simulink model "three_phase_squirrel_machine"  (R2017a)
settings: Solver=ode23tb  StartTime=0.0  StopTime=16  FixedStep=0.001  MaxStep=1e-4  MinStep=1e-7  RelTol=1e-3  AbsTol=.05  EnableMultiTasking=on
libraries: powerlib x17, simulink x1
settings Model: Creator=Administrator  LastModifiedBy=90584
settings DataIOCC: LimitDataPoints=on  SaveFormat=Array  SignalLoggingSaveFormat=ModelDataLogs
settings OptimizationCC: InitFltsAndDblsToZero=on  LifeSpan=inf
settings DebuggingCC: SaveWithParameterizedLinksMsg=none  UnderspecifiedInitializationDetection=Classic  MergeDetectMultiDrivingBlocksExec=none  SignalResolutionControl=TryResolveAllWithWarning  SolverPrmCheckMsg=warning  MultiTaskDSMMsg=warning  MultiTaskCondExecSysMsg=none  FcnCallInpInsideContextMsg=warning  SFUnexpectedBacktrackingDiag=warning  SFNoUnconditionalDefaultTransitionDiag=warning  SFExecutionAtInitializationDiag=none
settings HardwareCC: ProdBitPerPointer=32  ProdBitPerSizeT=32  ProdBitPerPtrDiffT=32  ProdLargestAtomicFloat=None  ProdIntDivRoundTo=Undefined  ProdEndianess=Unspecified  ProdWordSize=32  ProdHWDeviceType=32-bit Generic
settings ModelReferenceCC: PropagateSignalLabelsOutOfModel=off
settings GRTTargetCC: TargetFcnLib=ansi_tfl_tmw.mat  TargetLangStandard=C89/C90 (ANSI)  CombineOutputUpdateFcns=off  GRTInterface=on
settings ConfigComp: CovMetricSettings=dw  CovHtmlReporting=on  CovSaveCumulativeToWorkspaceVar=on  CovSaveSingleToWorkspaceVar=on  CovExternalEMLEnable=off

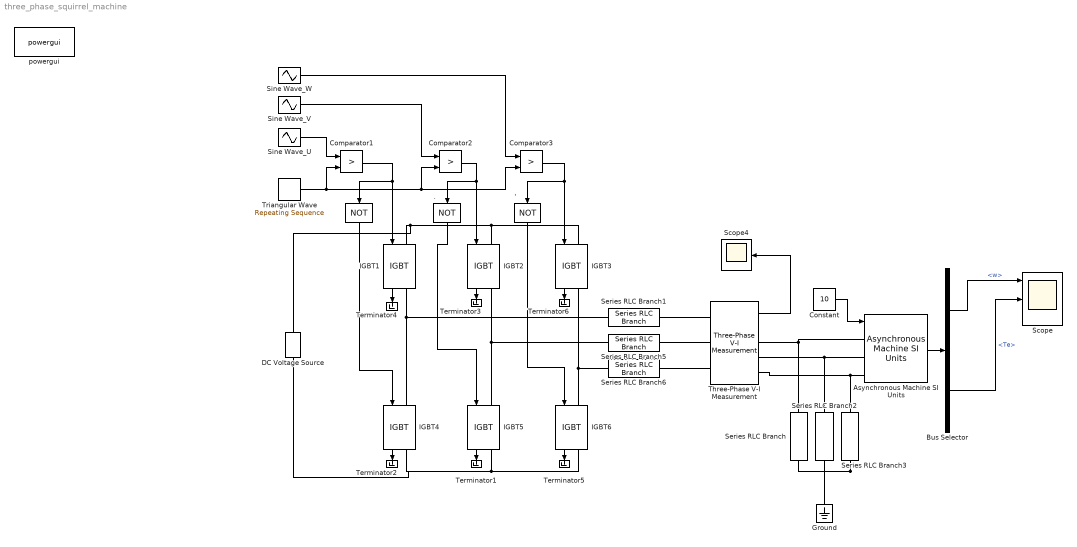
== system three_phase_squirrel_machine ==
  " " : Logic  Operator=NOT  AllPortsSameDT=off  OutDataTypeStr=boolean
  " '" : Logic  Operator=NOT  AllPortsSameDT=off  OutDataTypeStr=boolean
  " ." : Logic  Operator=NOT  AllPortsSameDT=off  OutDataTypeStr=boolean
  Asynchronous Machine SI Units : powerlib/Machines/Asynchronous Machine SI Units  RotorType=Squirrel-cage  PresetModel=No  MechanicalLoad=Torque Tm  ShowDetailedParameters=on  ReferenceFrame=Stationary  Units=SI  MeasurementBus=on  NominalParameters=[3*800,110,50]  Stator=[0.635 1*2.0e-3]  Rotor=[0.816 1.5e-3]  Cage1=[0.4155 0.002066]  Cage2=[0.4168 0.0003495]  Lm=76.31e-3  Mechanical=[0.25 0 2]  PolePairs=2  InitialConditions=[1 0 0 0 0 0 0 0]  SimulateSaturation=off  Saturation=[14.03593122, 27.81365428, 53.79336849, 72.68890987, 97.98006896, 148.6815601, 215.7428561, 302.9841135, 428.7778367 ; 230, 322, 414, 460, 506, 552, 598, 644, 690]  LoadFlowParameters=1492000  TsPowergui=0  TsBlock=-1  IterativeModel=Trapezoidal non iterative  IterativeDiscreteModel=Trapezoidal non iterative  Pmec=1.492e+006
  Bus Selector : BusSelector  OutputSignals=w,Te
  Comparator1 : RelationalOperator  Operator=>  OutDataTypeStr=boolean  RndMeth=Nearest
  Comparator2 : RelationalOperator  Operator=>  OutDataTypeStr=boolean  RndMeth=Nearest
  Comparator3 : RelationalOperator  Operator=>  OutDataTypeStr=boolean  RndMeth=Nearest
  Constant : Constant  Value=10
  DC Voltage Source : powerlib/Electrical Sources/DC Voltage Source  Amplitude=50  Measurements=None
  Ground : powerlib/Elements/Ground  LConnTagsString=a
  IGBT{1..6} (6 alike) : powerlib/Power Electronics/IGBT  Ron=0.001  Lon=0  Vf=1  Tf=1e-6  Tt=2e-6  IC=0  Rs=1e5  Cs=inf  Measurements=on
  Scope : Scope  NumInputPorts=3
  Scope4 : Scope
  Series RLC Branch : powerlib/Elements/Series RLC Branch  LConnTagsString=__new0  RConnTagsString=__new0  BranchType=C  Resistance=1  Inductance=1e-3  SetiL0=off  InitialCurrent=0  Capacitance=1e-3  Setx0=off  InitialVoltage=0  Measurements=None
  Series RLC Branch1 : powerlib/Elements/Series RLC Branch  LConnTagsString=__new0  RConnTagsString=__new0  BranchType=L  Resistance=1  Inductance=1e-3  SetiL0=off  InitialCurrent=0  Capacitance=1e-3  Setx0=off  InitialVoltage=0  Measurements=None
  Series RLC Branch2 : powerlib/Elements/Series RLC Branch  LConnTagsString=__new0  RConnTagsString=__new0  BranchType=C  Resistance=1  Inductance=1e-3  SetiL0=off  InitialCurrent=0  Capacitance=1e-3  Setx0=off  InitialVoltage=0  Measurements=None
  Series RLC Branch3 : powerlib/Elements/Series RLC Branch  LConnTagsString=__new0  RConnTagsString=__new0  BranchType=C  Resistance=1  Inductance=1e-3  SetiL0=off  InitialCurrent=0  Capacitance=1e-3  Setx0=off  InitialVoltage=0  Measurements=None
  Series RLC Branch5 : powerlib/Elements/Series RLC Branch  LConnTagsString=__new0  RConnTagsString=__new0  BranchType=L  Resistance=1  Inductance=1e-3  SetiL0=off  InitialCurrent=0  Capacitance=1e-3  Setx0=off  InitialVoltage=0  Measurements=None
  Series RLC Branch6 : powerlib/Elements/Series RLC Branch  LConnTagsString=__new0  RConnTagsString=__new0  BranchType=L  Resistance=1  Inductance=1e-3  SetiL0=off  InitialCurrent=0  Capacitance=1e-3  Setx0=off  InitialVoltage=0  Measurements=None
  Sine Wave_U : Sin  Amplitude=0.7  Frequency=188.4956/2  SampleTime=0
  Sine Wave_V : Sin  Amplitude=0.7  Frequency=188.4956/2  Phase=-2*pi/3  SampleTime=0
  Sine Wave_W : Sin  Amplitude=0.7  Frequency=188.4956/2  Phase=2*pi/3  SampleTime=0
  Terminator{1..6} (6 alike) : Terminator
  Three-Phase V-I Measurement : powerlib/Measurements/Three-Phase V-I Measurement  VoltageMeasurement=phase-to-ground  SetLabelV=off  LabelV=Vabc  Vpu=off  VpuLL=off  CurrentMeasurement=yes  SetLabelI=off  LabelI=Iabc  Ipu=off  Pbase=100e6  Vbase=500e3  OutputType=Complex  PhasorSimulation=off  PSBequivalent=0
  Triangular Wave : simulink/Sources/Repeating Sequence  rep_seq_t=[0 2.5e-5 5e-5 7.5e-5 1e-4]  rep_seq_y=[0 1 0 -1 0]
  powergui : powerlib/powergui  Priority=1  SimulationMode=Discrete  SampleTime=1e-6  frequency=60  Iterations=50  frequencyindice=0  Pbase=100e6  ErrMax=1e-4  UnitsV=kV  UnitsW=MW  buscounter=0  FunctionMessages=off  echomessages=off  EnableUseOfTLC=off  CurrentSourceSwitches=off  DisableSnubberDevices=off  DisableRonSwitches=off  DisableVfSwitches=off  DisplayEquations=off  SolverType=Tustin/Backward Euler (TBE)  Interpol=off  ExternalGateDelay=off  methode=off  Ts=100  x0status=blocks  SPID=on  SwTol=0  HookPort=off  RestoreLinks=warning  ResistiveCurrentMeasurement=off  Frange=[0:2:500]  Ylog=off  Xlog=on  ShowGrid=off  save=off  variable=ZData  structure=0  ZoomFFT=off  StartTime=0.0  cycles=1  DisplayStyle=1  fundamental=60  FreqAxis=off  MaxFrequency=1000  frequencyindicesteady=1  RmsSteady=1  display=off
  wires:
  Sine Wave_V/1 -> Comparator2/1
  Comparator1/1 -> IGBT1/1, " "/1
  IGBT2/1 -> Terminator3/1
  Triangular Wave/1 -> Comparator1/2, Comparator2/2, Comparator3/2
  Comparator2/1 -> IGBT2/1, " ."/1
  IGBT1/1 -> Terminator4/1
  " '"/1 -> IGBT6/1
  Sine Wave_W/1 -> Comparator3/1
  IGBT5/1 -> Terminator1/1
  Comparator3/1 -> IGBT3/1, " '"/1
  Sine Wave_U/1 -> Comparator1/1
  " "/1 -> IGBT4/1
  " ."/1 -> IGBT5/1
  IGBT3/1 -> Terminator6/1
  IGBT4/1 -> Terminator2/1
  IGBT6/1 -> Terminator5/1
  Bus Selector/1 -> Scope/1  "<w>"
  Asynchronous Machine SI Units/1 -> Bus Selector/1
  Constant/1 -> Asynchronous Machine SI Units/1
  Three-Phase V-I Measurement/1 -> Scope4/1
  Bus Selector/2 -> Scope/2  "<Te>"
  connections:
  IGBT6/LConn1 -- IGBT3/RConn1 -- Series RLC Branch6/RConn1
  IGBT2/RConn1 -- Series RLC Branch5/RConn1 -- IGBT5/LConn1
  IGBT4/LConn1 -- IGBT1/RConn1 -- Series RLC Branch1/RConn1
  IGBT5/RConn1 -- DC Voltage Source/LConn1 -- IGBT4/RConn1 -- IGBT6/RConn1
  IGBT1/LConn1 -- DC Voltage Source/RConn1 -- IGBT3/LConn1 -- IGBT2/LConn1
  Series RLC Branch/LConn1 -- Three-Phase V-I Measurement/RConn1 -- Asynchronous Machine SI Units/LConn1
  Series RLC Branch2/LConn1 -- Three-Phase V-I Measurement/RConn2 -- Asynchronous Machine SI Units/LConn2
  Series RLC Branch3/LConn1 -- Three-Phase V-I Measurement/RConn3 -- Asynchronous Machine SI Units/LConn3
  Series RLC Branch3/RConn1 -- Ground/LConn1 -- Series RLC Branch/RConn1 -- Series RLC Branch2/RConn1
  Series RLC Branch1/LConn1 -- Three-Phase V-I Measurement/LConn1
  Series RLC Branch5/LConn1 -- Three-Phase V-I Measurement/LConn2
  Series RLC Branch6/LConn1 -- Three-Phase V-I Measurement/LConn3
